simulink model "Sim3dot0"  (R2023b)
settings: Solver=VariableStepAuto  StartTime=0.0  StopTime=10.0  RelTol=1e-3
values from neighbouring files (symbols this model uses):
  cg_z = 0.335    [para_sim1dot4.mat]    (also in para_sim1dot5.mat; para_sim1dot6.mat = 0.215; para_sim1dot7.mat = 0.215)
  dt = 0.02    [para_sim1dot0.mat]    (also in para_sim1dot1.mat; para_sim1dot2.mat; para_sim1dot3.mat; para_sim1dot4.mat)
  F35thrust = [0 0.011 0.018 0.024 0.031 0.037 0.046 0.053 0.061 0.07 0.079 0.088 ... (170 elements, 85x2)]    [para_sim1dot3.mat]    (also in para_sim1dot4.mat; para_sim1dot5.mat; para_sim1dot6.mat; para_sim1dot7.mat)
  fin_drag_over_v2 = [-30 -25 -20 -15 -10 -5 0 5 10 15 20 25 ... (26 elements, 13x2)]    [para_sim1dot2.mat]    (also in para_sim1dot3.mat; para_sim1dot4.mat; para_sim1dot5.mat; para_sim1dot6.mat)
  fin_lift_over_v2 = [-30 -25 -20 -15 -10 -5 0 5 10 15 20 25 ... (26 elements, 13x2)]    [para_sim1dot2.mat]    (also in para_sim1dot3.mat; para_sim1dot4.mat; para_sim1dot5.mat; para_sim1dot6.mat)
  l_arm_moment = 0.5    [para_sim1dot2.mat]    (also in para_sim1dot3.mat; para_sim1dot4.mat = 0.3; para_sim1dot5.mat = 0.3; para_sim1dot6.mat = 0.175)
  mass = 1    [para_sim1dot0.mat]    (also in para_sim1dot1.mat; para_sim1dot2.mat = 0.6; para_sim1dot3.mat = 0.8; para_sim1dot4.mat = 0.8)
  max_fin_angle_deg = 30    [para_sim1dot0.mat]    (also in para_sim1dot1.mat; para_sim1dot2.mat; para_sim1dot3.mat; para_sim1dot4.mat)
  r_arm_moment = 0.05    [para_sim1dot2.mat]    (also in para_sim1dot3.mat; para_sim1dot4.mat; para_sim1dot5.mat; para_sim1dot6.mat = 0.065)
  servo_slew_radps = 5.23    [para_sim1dot5.mat]    (also in para_sim1dot6.mat; para_sim1dot7.mat)
libraries: simulink_extras x16, slpidlib x6, shared6dof x1, matrix_library x1, sharedtransform x1, aerolibanimutils x1, uavutilslib x1
(part 2 of 2)

== matlab function Sim3dot0/Fin effects/2D Coord transform from wind to body sys2 ==
  data: vec_in input; vec_out output; gamma input
function vec_out = wind2body_fin(vec_in, gamma) % beta converts vec in wind sys to 0 fin angle sys which is parallel to rocket body sys

vec_in_T = transpose(vec_in);
vec_out = [1, 0,         0;
           0, cos(gamma), -sin(gamma);
           0, sin(gamma), cos(gamma),] * vec_in_T;

== matlab function Sim3dot0/Fin effects/2D Coord transform from wind to body sys3 ==
  data: vec_in input; vec_out output; gamma input
function vec_out = wind2body_fin(vec_in, gamma) % beta converts vec in wind sys to 0 fin angle sys which is parallel to rocket body sys

vec_in_T = transpose(vec_in);
vec_out = [1, 0,         0;
           0, cos(gamma), -sin(gamma);
           0, sin(gamma), cos(gamma),] * vec_in_T;

== matlab function Sim3dot0/Matlab sys to user sys4 ==
  data: M_dcm input; M_6dof output
function M_6dof = fcn(M_dcm)
M_lab2user = [0 1 0; 1 0 0; 0 0 -1];
M_6dof = M_lab2user * M_dcm;

== matlab function Sim3dot0/Matlab sys to user sys7 ==
  data: M_dcm input; M_6dof output
function M_6dof = fcn(M_dcm)
M_lab2user = [0 1 0; 1 0 0; 0 0 -1];
M_6dof = M_lab2user * M_dcm;

== matlab function Sim3dot0/Matlab sys to user sys8 ==
  data: M_dcm input; M_6dof output
function M_6dof = fcn(M_dcm)
M_lab2user = [0 1 0; 1 0 0; 0 0 -1];
M_6dof = M_lab2user * M_dcm;

== matlab function Sim3dot0/MATLAB Function2 ==
  data: output_x_pitch input; ang1 output; output_y_roll input; output_z_yaw input; ang2 output; ang3 output; ang4 output
function [ang1, ang2, ang3, ang4] = control2fin(output_x_pitch, output_y_roll, output_z_yaw)

ang1 = (output_z_yaw + 0. + output_x_pitch);
ang2 = (output_z_yaw + output_y_roll + 0.);
ang3 = (output_z_yaw + 0. - output_x_pitch);
ang4 = (output_z_yaw - output_y_roll + 0.);

== matlab function Sim3dot0/Matlab sys to user sys9 ==
  data: M_dcm input; M_6dof output
function M_6dof = fcn(M_dcm)
M_lab2user = [0 1 0; 1 0 0; 0 0 -1];
M_6dof = M_lab2user * M_dcm;

== matlab function Sim3dot0/MATLAB Function4 ==
  data: pos_z input; stop output
function stop = alt_stop(pos_z)
if pos_z < -1
    stop = 1;
else
    stop = 0;
end

== matlab function Sim3dot0/Matlab sys to user sys1 ==
  data: M_dcm input; M_6dof output
function M_6dof = fcn(M_dcm)
M_lab2user = [0 1 0; 1 0 0; 0 0 -1];
M_6dof = M_lab2user * M_dcm;

== matlab function Sim3dot0/MATLAB Function5 ==
  settings: updateMethod=DISCRETE
  data: in input; out output
function out = run_max(in)
persistent max_old

if isempty(max_old)
    out = in;
    max_old = in;
else
    if in > max_old
        out = in;
        max_old = in;
    else
        out = max_old;
    end
end

== matlab function Sim3dot0/Launch rail model/MATLAB Function7 ==
  data: real_moment input; out_moment output; z_alt input; h_rail input
function out_moment = launch_rod_go_straight_M(real_moment, z_alt, h_rail)
if z_alt >= h_rail
    out_moment = real_moment;
else
    out_moment = [0 0 0];
end

== matlab function Sim3dot0/Launch rail model1/MATLAB Function7 ==
  data: real_force input; out_force output; z_alt input; h_rail input
function out_force = launch_rod_go_straight_F(real_force, z_alt, h_rail)
if z_alt >= h_rail
    out_force = real_force;
else
    out_force = [0 0 real_force(3)];
end

== matlab function Sim3dot0/Matlab sys to user sys3 ==
  data: M_dcm input; M_6dof output
function M_6dof = fcn(M_dcm)
M_lab2user = [0 1 0; 1 0 0; 0 0 -1];
M_6dof = M_lab2user * M_dcm;

== matlab function Sim3dot0/M: Fin to body sys ==
  data: fin1 input; vec output; fin2 input; fin3 input; fin4 input
function vec = fcn(fin1, fin2, fin3, fin4)
vx = -fin1 + fin3; % CW moment is positive, in negative x dir
vy = -fin2 + fin4;
vz = 0;

vec = [vx, vy, vz];

== matlab function Sim3dot0/Fin effects/M: Force induced moments on body ==
  data: F1 input; M output; F2 input; F3 input; F4 input; r_arm_moment input; l_arm_moment input
function M = fcn(F1, F2, F3, F4, r_arm_moment, l_arm_moment)

r1 = [r_arm_moment, 0, -l_arm_moment];
r2 = [0, r_arm_moment, -l_arm_moment];
r3 = [-r_arm_moment, 0, -l_arm_moment];
r4 = [0, -r_arm_moment, -l_arm_moment];

F1_body = F1;
F2_body = [-F2(2) F2(1) F2(3)];
F3_body = [-F3(1) -F3(2) F3(3)];
F4_body = [F4(2) -F4(1) F4(3)];
M = cross(r1, F1_body) + cross(r2, F2_body) + cross(r3, F3_body) + cross(r4, F4_body);

== matlab function Sim3dot0/Fin effects/Convert fin lift drag to  ==
  data: cl_arr input; F1 output; cd_arr input; F2 output; F3 output; F4 output
function [F1, F2, F3, F4]= fcn(cl_arr, cd_arr)
F1 = [0, cl_arr(1), -cd_arr(1)];
F2 = [0, cl_arr(2), -cd_arr(2)];
F3 = [0, cl_arr(3), -cd_arr(3)];
F4 = [0, cl_arr(4), -cd_arr(4)];

== matlab function Sim3dot0/User sys to Matlab sys2 ==
  data: M_me input; M_6dof output
function M_6dof = fcn(M_me)
M_6dof = [M_me(2), M_me(1), -M_me(3)];

== matlab function Sim3dot0/User sys to Matlab sys1 ==
  data: M_me input; M_6dof output
function M_6dof = fcn(M_me)
M_6dof = [M_me(2), M_me(1), -M_me(3)];

== matlab function Sim3dot0/V air: Body to fin sys1 ==
  data: v_air_b input; v_f1 output; v_f2 output; v_f3 output; v_f4 output
function [v_f1, v_f2, v_f3, v_f4]= fcn(v_air_b)
vx = v_air_b(1);
vy = v_air_b(2);
vz = v_air_b(3);

v_f1 = [vx, vy, vz];
v_f2 = [vy, -vx, vz];
v_f3 = [-vx, -vy, vz];
v_f4 = [-vy, vx, vz];

== matlab function Sim3dot0/Matlab sys to user sys ==
  data: M_dcm input; M_6dof output
function M_6dof = fcn(M_dcm)
M_lab2user = [0 1 0; 1 0 0; 0 0 -1];
M_6dof = M_lab2user * M_dcm;

== matlab function Sim3dot0/Matlab sys to user sys2 ==
  data: M_dcm input; M_6dof output
function M_6dof = fcn(M_dcm)
M_lab2user = [0 1 0; 1 0 0; 0 0 -1];
M_6dof = M_lab2user * M_dcm;
